simulink model "ConstructionCradleControl"  (R2023a)
settings: Solver=ode15s  StartTime=0.0  StopTime=10  FixedStep=1e-3  RelTol=1e-3
values from neighbouring files (symbols this model uses):
  kd = 0.0824380679349514    (= 0.082438067935)    [PID_coef.m]
  ki = 0.12628634535922    (= 0.126286345359)    [PID_coef.m]
  kp = 115.072226705239    (= 115.072226705)    [PID_coef.m]
settings Model: Creator=Ilya_Andriyanov  LastModifiedBy=ПК

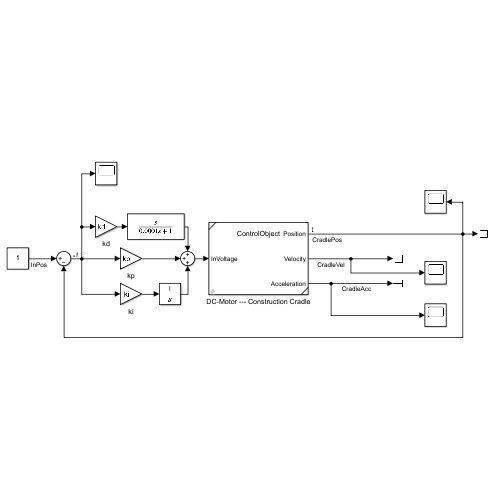
[thumbnail: Simulink's stored preview of the top-level diagram]
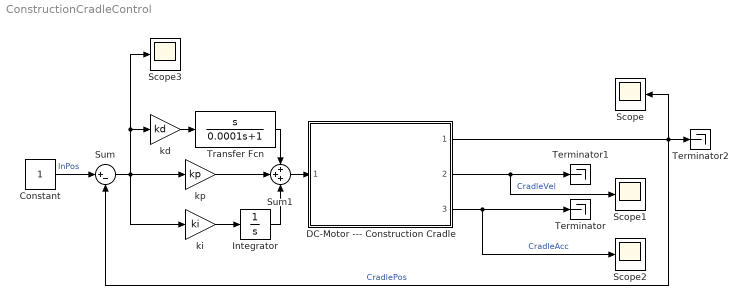
== system ConstructionCradleControl ==
  Constant : Constant
  DC-Motor --- Construction Cradle : Subsystem  ReferencedSubsystem=ControlObject  motor_nominal_voltage=24  L=300e-6  R=8.5  km=17e-1  kw=17e-2  J_motor=500e-9  vis_friction_coef_motor=0.001  i_gear=200  J_gear=2.4e-9  vis_friction_coef_gear=0.001  r_cyl=0.3  vis_friction_coef_cradle=0.001  cradle_mass=10
  Integrator : Integrator
  Scope{,1..3} (4 alike) : Scope
  Sum : Sum  Inputs=|+-
  Sum1 : Sum  Inputs=+++
  Terminator : Terminator
  Terminator1 : Terminator
  Terminator2 : Terminator
  Transfer Fcn : TransferFcn  Numerator=[1 0]  Denominator=[0.0001 1]
  kd : Gain  Gain=kd
  ki : Gain  Gain=ki
  kp : Gain  Gain=kp
  wires:
  DC-Motor --- Construction Cradle/2 -> Scope1/1, Terminator1/1  "CradleVel"
  DC-Motor --- Construction Cradle/3 -> Scope2/1, Terminator/1  "CradleAcc"
  Constant/1 -> Sum/1  "InPos"
  kd/1 -> Transfer Fcn/1
  Transfer Fcn/1 -> Sum1/1
  kp/1 -> Sum1/2
  ki/1 -> Integrator/1
  Integrator/1 -> Sum1/3
  DC-Motor --- Construction Cradle/1 -> Terminator2/1, Scope/1, Sum/2  "CradlePos"
  Sum1/1 -> DC-Motor --- Construction Cradle/1
  Sum/1 -> kd/1, Scope3/1, kp/1, ki/1
